simulink model "Coupled3DPathFollowing"  (R2024a)
settings: Solver=ode4  StartTime=0.0  StopTime=inf  FixedStep=0.05  RelTol=1e-3
InitFcn:
  | initModelParam;
  | SetWaypoints;
StopFcn:
  | plotCoupled3DTrack;
values from neighbouring files (symbols this model uses):
  Waypoints = [20 32.5 45 57.5 70 40 63.75 87.5 111.25 135 10 11.25 ... (15 elements, 5x3)]    [Waypoints.mat]
undefined symbols (not defined in the file or in its folder): P0, WPNum
libraries: slpidlib x2, simulink x1, vrlib x1
settings Model: Creator=53549  LastModifiedBy=kedarpandya
settings SolverCC: AlgebraicLoopSolver=TrustRegion
settings DataIOCC: ReturnWorkspaceOutputs=off
settings DebuggingCC: UnconnectedInputMsg=warning  UnconnectedOutputMsg=warning  UnconnectedLineMsg=warning  ArithmeticOperatorsInVariantConditions=warning
settings ModelReferenceCC: EnableRefExpFcnMdlSchedulingChecks=on
settings SFSimCC: SimUseLocalCustomCode=off  CustomCodeUndefinedFunction=UseInterfaceOnly
settings RTWCC: RTWUseLocalCustomCode=off  GPUComputeCapability=3.5  DLArmComputeVersion=19.05
settings CodeAppCC: StateflowObjectComments=on

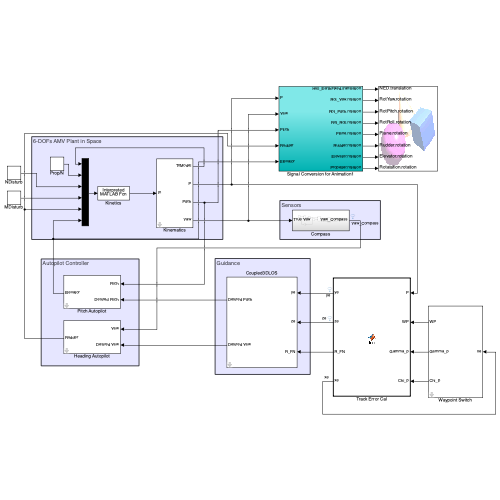
[thumbnail: Simulink's stored preview of the top-level diagram]
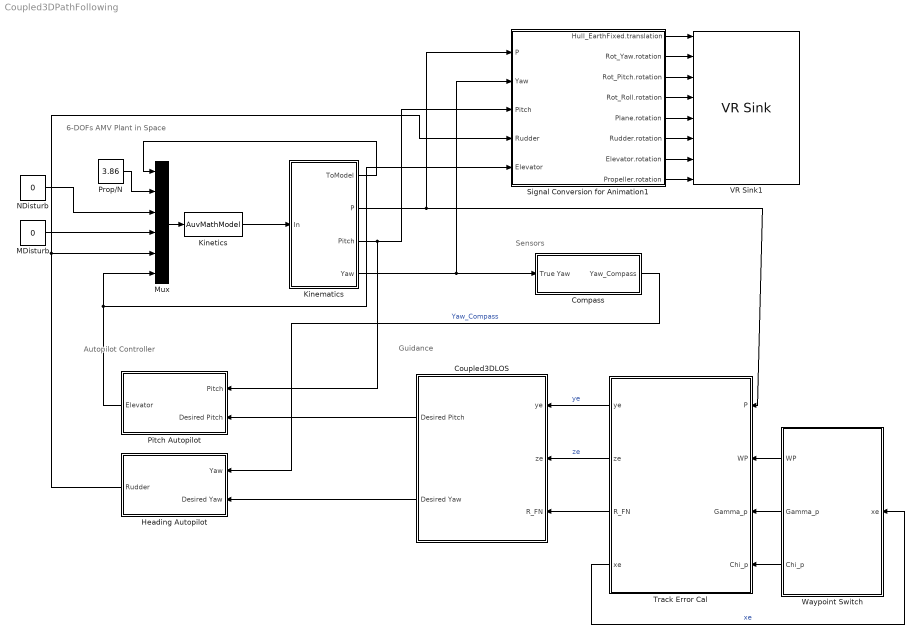
== system Coupled3DPathFollowing ==
  note: Sensors
  note: Guidance
  note: Autopilot Controller
  note: 6-DOFs AMV Plant in Space
  Compass : Subsystem
  Coupled3DLOS : Subsystem  mask{LOSAlg=ALOS, Delta=3, Kapa=0.1, Gamma=0.15}
      mask prompts: LOSAlg "制导算法"; Delta "前视距离"; Kapa "漂角自适应估计增益"; Gamma "攻角自适应估计增益"
      mask TypeOptions LOSAlg: LOS | ALOS
      mask DialogControl DescGroupVar Prompt: 三维视线角制导
      mask DialogControl DescTextVar Prompt: 设置三维视线角制导参数：前视距离，漂角自适应估计增益，漂角自适应估计增益。自适应估计增益设置为0，屏蔽估计补偿；非0，启用估计补偿。
      mask DialogControl Container5 Prompt: 旋转制导算法
      mask DialogControl ParameterGroupVar Prompt: 设置制导参数
  Heading Autopilot : Subsystem  mask{kp=1, ki=0, kd=1.5}
      mask DialogControl DescGroupVar Prompt: Heading Autopilot
      mask DialogControl DescTextVar Prompt: 设置PID增益。
      mask DialogControl ParameterGroupVar Prompt: PID Parameter
  Kinematics : Subsystem  mask{x0=0, y0=0, z0=0.2, pitch0=0, yaw0=68.5, u0=0.6, flowDir=45, flowVel=0.1}
      mask prompts: x0 "Initiral x"; y0 "Initiral y"; z0 "Initiral z"; pitch0 "Initial pitch [Deg]"; yaw0 "Initial yaw [Deg]"; u0 "Initial velocity [m/s]"; flowDir "Flow direction [Deg]"; flowVel "Flow velocity [m/s]"
      mask DialogControl DescGroupVar Prompt: Kinematics
      mask DialogControl DescTextVar Prompt: Set kinematics information: AMV initial state, flow interference, etc
      mask DialogControl ParameterGroupVar Prompt: Initial state
      mask DialogControl Container3 Prompt: Flow
  Kinetics : MATLABFcn  MATLABFcn=AuvMathModel  OutputDimensions=6  OutputSignalType=real
  MDisturb : Constant  Value=0
  Mux : Mux  Inputs=6
  NDisturb : Constant  Value=0
  Pitch Autopilot : Subsystem  mask{kp=2, ki=0.5, kd=1.5}
      mask DialogControl DescGroupVar Prompt: Pitch Autopilot
      mask DialogControl DescTextVar Prompt: 设置PID控制增益。
      mask DialogControl ParameterGroupVar Prompt: PID Parameter
  Prop/N : Constant  Value=3.86
  Signal Conversion for Animation1 : Subsystem
  Track Error Cal : MATLAB Function  TreatAsAtomicUnit=on
  VR Sink1 : vrlib/VR Sink  InstantiateOnLoad=on  SampleTime=0.1  ViewEnable=on  RemoteChange=off  RemoteView=off  FieldsWritten=NED.translation.3.1.1.double#RotYaw.rotation.4.1.1.double#RotPitch.rotation.4.1.1.double#RotRoll.rotation.4.1.1.double#Plane.rotation.4.1.1.double#Rudder.rotation.4.1.1.double#Elevator.rotation.4.1.1.double#Rotatation.rotation.4.1.1.double  WorldFileName=SubMarine.wrl  AutoView=on  VideoDimensions=[]  AllowVariableSize=off  FigureProperties="{'Position', 'Name', 'Viewpoint', 'CameraBound', 'CameraDirection', 'CameraPosition', 'CameraUpVector', 'ZoomFactor', 'Antialiasing', 'Headlight', 'Lighting', 'Sound', 'StatusBar', 'Stereo3D', 'Stereo3DCameraOffset', 'Stereo3DHIT', 'ToolBar', 'Textures', 'Transparency', 'Triad', 'Wireframe', 'NavZones', 'NavMode', 'NavSpeed', 'CaptureFileFormat', 'CaptureFileName', 'Record2DCompressMethod', 'Record2DCompressQuality', 'Record2D', 'Record2DFileName', 'Record2DFPS', 'NavPanel'; [8.6000000000000000e+01   1.0300000000000000e+02   5.7600000000000000e+02   3.5000000000000000e+02], '', 'Stern', 'on', [0.0000000000000000e+00   0.0000000000000000e+00  -1.0000000000000000e+00], [0.0000000000000000e+00   0.0000000000000000e+00   0.0000000000000000e+00], [0.0000000000000000e+00   1.0000000000000000e+00   0.0000000000000000e+00], [1.0000000000000000e+00], 'on', 'on', 'on', 'on', 'on', 'off', [1.0000000149011612e-01], [0.0000000000000000e+00], 'on', 'on', 'on', 'none', 'off', 'off', 'fly', 'normal', 'tif', '%f_anim_%n.tif', 'auto', [7.5000000000000000e+01], 'off', '%f_anim_%n.avi', 'auto', 'halfbar'}"
  Waypoint Switch : Subsystem  mask{WP=Waypoints, WPNum=WPNum}
      mask prompts: WP "航点序列"; WPNum "航点个数"
      mask DialogControl DescGroupVar Prompt: 航点设置
      mask DialogControl DescTextVar Prompt: 设置航点序列和个数
  wires:
  Kinetics/1 -> Kinematics/1(In)
  Mux/1 -> Kinetics/1
  Kinematics/4(Yaw) -> Signal Conversion for Animation1/2(Yaw), Compass/1(True Yaw)
  Kinematics/1(ToModel) -> Mux/1
  Prop/N/1 -> Mux/2
  NDisturb/1 -> Mux/3
  Track Error Cal/4(xe) -> Waypoint Switch/1(xe)  "xe"
  Waypoint Switch/2(Gamma_p) -> Track Error Cal/3(Gamma_p)
  MDisturb/1 -> Mux/4
  Kinematics/2(P) -> Signal Conversion for Animation1/1(P), Track Error Cal/1(P)
  Kinematics/3(Pitch) -> Signal Conversion for Animation1/3(Pitch), Pitch Autopilot/1(Pitch)
  Waypoint Switch/3(Chi_p) -> Track Error Cal/4(Chi_p)
  Waypoint Switch/1(WP) -> Track Error Cal/2(WP)
  Track Error Cal/1(ye) -> Coupled3DLOS/1(ye)  "ye"
  Track Error Cal/2(ze) -> Coupled3DLOS/2(ze)  "ze"
  Track Error Cal/3(R_FN) -> Coupled3DLOS/3(R_FN)
  Coupled3DLOS/1(Desired Pitch) -> Pitch Autopilot/2(Desired Pitch)
  Coupled3DLOS/2(Desired Yaw) -> Heading Autopilot/2(Desired Yaw)
  Compass/1(Yaw_Compass) -> Heading Autopilot/1(Yaw)  "Yaw_Compass"
  Heading Autopilot/1(Rudder) -> Signal Conversion for Animation1/4(Rudder), Mux/5
  Pitch Autopilot/1(Elevator) -> Signal Conversion for Animation1/5(Elevator), Mux/6
  Signal Conversion for Animation1/1(Hull_EarthFixed.translation) -> VR Sink1/1
  Signal Conversion for Animation1/2(Rot_Yaw.rotation) -> VR Sink1/2
  Signal Conversion for Animation1/3(Rot_Pitch.rotation) -> VR Sink1/3
  Signal Conversion for Animation1/4(Rot_Roll.rotation) -> VR Sink1/4
  Signal Conversion for Animation1/5(Plane.rotation) -> VR Sink1/5
  Signal Conversion for Animation1/8(Propeller.rotation) -> VR Sink1/8
  Signal Conversion for Animation1/6(Rudder.rotation) -> VR Sink1/6
  Signal Conversion for Animation1/7(Elevator.rotation) -> VR Sink1/7

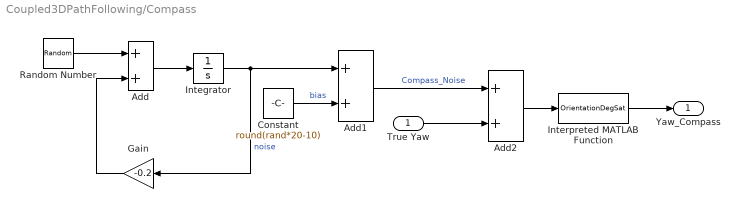
== system Coupled3DPathFollowing/Compass ==
  True Yaw : Inport
  Add : Sum
  Add1 : Sum
  Add2 : Sum
  Constant : Constant  Value=round(rand*20-10)
  Gain : Gain  Gain=-0.2
  Integrator : Integrator
  Interpreted MATLAB Function : MATLABFcn  MATLABFcn=OrientationDegSat
  Random Number : RandomNumber  Variance=0.05  Seed=round(rand*20)  SampleTime=1
  Yaw_Compass : Outport
  wires:
  Constant/1 -> Add1/2  "bias"
  Random Number/1 -> Add/1
  Integrator/1 -> Add1/1, Gain/1  "noise"
  Gain/1 -> Add/2
  Add/1 -> Integrator/1
  Add1/1 -> Add2/1  "Compass_Noise"
  True Yaw/1 -> Add2/2
  Interpreted MATLAB Function/1 -> Yaw_Compass/1
  Add2/1 -> Interpreted MATLAB Function/1

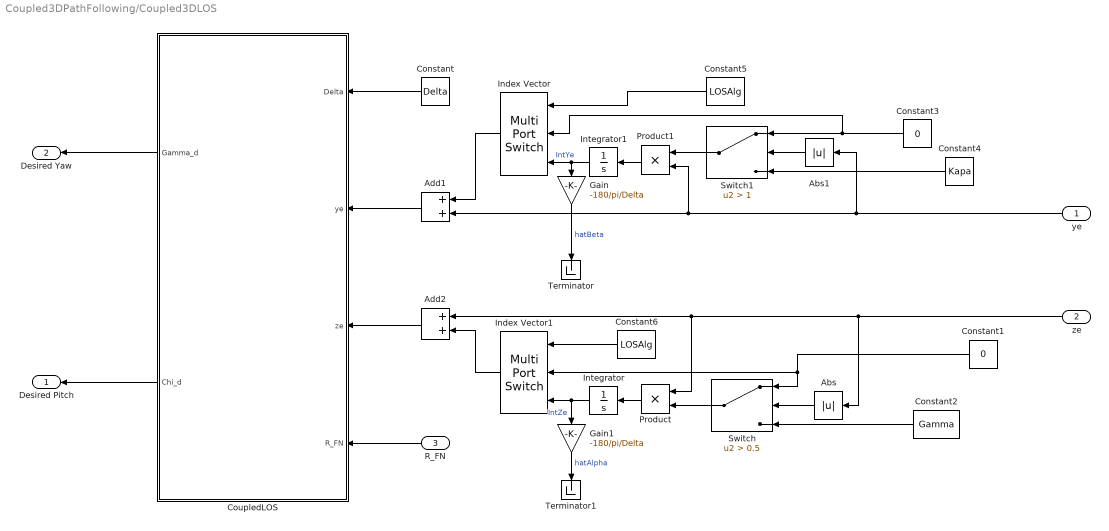
== system Coupled3DPathFollowing/Coupled3DLOS ==
  ye : Inport
  ze : Inport  Port=2
  R_FN : Inport  Port=3
  Abs : Abs  SaturateOnIntegerOverflow=off
  Abs1 : Abs  SaturateOnIntegerOverflow=off
  Add1 : Sum
  Add2 : Sum
  Constant : Constant  Value=Delta
  Constant1 : Constant  Value=0
  Constant2 : Constant  Value=Gamma
  Constant3 : Constant  Value=0
  Constant4 : Constant  Value=Kapa
  Constant5 : Constant  Value=LOSAlg
  Constant6 : Constant  Value=LOSAlg
  CoupledLOS : MATLAB Function  TreatAsAtomicUnit=on
  Gain : Gain  Gain=-180/pi/Delta
  Gain1 : Gain  Gain=-180/pi/Delta
  Index Vector : MultiPortSwitch  Inputs=2  SaturateOnIntegerOverflow=off  InputSameDT=off
  Index Vector1 : MultiPortSwitch  Inputs=2  SaturateOnIntegerOverflow=off  InputSameDT=off
  Integrator : Integrator
  Integrator1 : Integrator
  Product : Product
  Product1 : Product
  Switch : Switch  Criteria=u2 > Threshold  Threshold=0.5  SaturateOnIntegerOverflow=off  InputSameDT=off
  Switch1 : Switch  Criteria=u2 > Threshold  Threshold=1  SaturateOnIntegerOverflow=off  InputSameDT=off
  Terminator : Terminator
  Terminator1 : Terminator
  Desired Pitch : Outport
  Desired Yaw : Outport  Port=2
  wires:
  Abs1/1 -> Switch1/2
  ze/1 -> Abs/1, Add2/1, Product/1
  Constant2/1 -> Switch/3
  Abs/1 -> Switch/2
  Product/1 -> Integrator/1
  Constant4/1 -> Switch1/3
  Constant1/1 -> Index Vector1/2, Switch/1
  ye/1 -> Add1/2, Product1/2, Abs1/1
  Integrator/1 -> Gain1/1, Index Vector1/3  "IntZe"
  Add2/1 -> CoupledLOS/3(ze)
  Product1/1 -> Integrator1/1
  Switch/1 -> Product/2
  Constant/1 -> CoupledLOS/1(Delta)
  CoupledLOS/2(Chi_d) -> Desired Pitch/1
  Switch1/1 -> Product1/1
  Constant3/1 -> Index Vector/2, Switch1/1
  Add1/1 -> CoupledLOS/2(ye)
  CoupledLOS/1(Gamma_d) -> Desired Yaw/1
  Integrator1/1 -> Gain/1, Index Vector/3  "IntYe"
  R_FN/1 -> CoupledLOS/4(R_FN)
  Constant5/1 -> Index Vector/1
  Index Vector/1 -> Add1/1
  Constant6/1 -> Index Vector1/1
  Index Vector1/1 -> Add2/2
  Gain/1 -> Terminator/1  "hatBeta"
  Gain1/1 -> Terminator1/1  "hatAlpha"

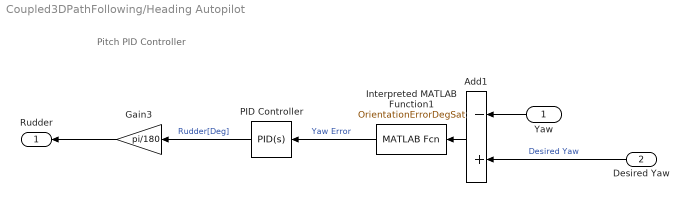
== system Coupled3DPathFollowing/Heading Autopilot ==
  note: Pitch PID Controller
  Yaw : Inport
  Desired Yaw : Inport  Port=2
  Add1 : Sum  Inputs=-+
  Gain3 : Gain  Gain=pi/180
  Interpreted MATLAB Function1 : MATLABFcn  MATLABFcn=OrientationErrorDegSat  OutputDimensions=1
  PID Controller : slpidlib/PID Controller  Controller=PID  Form=Parallel  TimeDomain=Continuous-time  UseExternalTs=off  SampleTime=-1  IntegratorMethod=Forward Euler  FilterMethod=Forward Euler  ControllerParametersSource=internal  P=kp  I=ki  UseKiTs=off  D=kd  UseExternalDerivativeSource=off  N=10  UseFilter=on  TunerSelectOption=Transfer Function Based (PID Tuner App)  InitialConditionSource=internal  InitialConditionForIntegrator=0  InitialConditionForFilter=0  DifferentiatorICPrevScaledInput=0  ExternalReset=none  TrackingMode=off  Kt=1  LimitOutput=on  SatLimitsSource=internal  UpperSaturationLimit=30  LowerSaturationLimit=-30  LinearizeAsGain=on  AntiWindupMode=none  Kb=1  LimitIntegrator=off  UpperIntegratorSaturationLimit=inf  LowerIntegratorSaturationLimit=-inf  POutMin=[]  POutMax=[]  IOutMin=[]  IOutMax=[]  DOutMin=[]  DOutMax=[]  NOutMin=[]  NOutMax=[]  SumOutMin=[]  SumOutMax=[]  SaturationOutMin=[]  SaturationOutMax=[]  PParamMin=[]  PParamMax=[]  IParamMin=[]  IParamMax=[]  DParamMin=[]  DParamMax=[]  NParamMin=[]  NParamMax=[]  KbParamMin=[]  KbParamMax=[]  KtParamMin=[]  KtParamMax=[]  KbOutMin=[]  KbOutMax=[]  KtOutMin=[]  KtOutMax=[]  IntegratorOutMin=[]  IntegratorOutMax=[]  FilterOutMin=[]  FilterOutMax=[]  SumI1OutMin=[]  SumI1OutMax=[]  SumI2OutMin=[]  SumI2OutMax=[]  SumI3OutMin=[]  SumI3OutMax=[]  SumI4OutMin=[]  SumI4OutMax=[]  SumDOutMin=[]  SumDOutMax=[]  DifferentiatorOutMin=[]  DifferentiatorOutMax=[]  FilterDiffOutCoefMin=[]  FilterDiffOutCoefMax=[]  ReciprocalOutMin=[]  ReciprocalOutMax=[]  SumDenOutMin=[]  SumDenOutMax=[]  SumNumOutMin=[]  SumNumOutMax=[]  DivideOutMin=[]  DivideOutMax=[]  UdiffTsProdOutMin=[]  UdiffTsProdOutMax=[]  NTsProdOutMin=[]  NTsProdOutMax=[]  UintegralTsProdOutMin=[]  UintegralTsProdOutMax=[]  UngainTsProdOutMin=[]  UngainTsProdOutMax=[]  ClampingZeroOutDataTypeStr=Inherit: Inherit via back propagation  ClampingZeroOutMin=[]  ClampingZeroOutMax=[]  FilterDenConstantOutDataTypeStr=Inherit: Inherit via back propagation  FilterDenConstantOutMin=[]  FilterDenConstantOutMax=[]  PCopyOutDataTypeStr=Inherit: Inherit via back propagation  PCopyOutMin=[]  PCopyOutMax=[]  NCopyOutDataTypeStr=Inherit: Inherit via back propagation  NCopyOutMin=[]  NCopyOutMax=[]  IntegratorContinuousStateAttributes=''  IntegratorStateMustResolveToSignalObject=off  IntegratorRTWStateStorageClass=Auto  FilterContinuousStateAttributes=''  FilterStateMustResolveToSignalObject=off  FilterRTWStateStorageClass=Auto  ParallelPVariant=InternalParameters  IdealPVariant=Disabled  IVariant=InternalParameters  DVariant=InternalParameters  IntegratorVariant=Continuous  SatVariant=Enabled  AWVariant=Passthrough  PCopyVariant=Disabled  TRVariant=Disabled  FdbkBlocksVariant=Forward  IdealPFdbkVariant=Disabled  SatFdbkVariant=Disabled  DerivativeFilterVariant=ContFilter  NVariant=InternalParameters  NCopyVariant=Disabled  FilterICVariant=InternalICsFilter  IntegratorICVariant=InternalICs  ExternalResetVariant=Disabled  TRSumVariant=Passthrough  SumFdbkVariant=Disabled  SumVariant=Sum_PID  TsampFilterVariant=InternalTs  TsampNgainVariant=Passthrough  TsampIntegralVariant=Disabled_SignalSpec  ExternalSaturationOutDataTypeStr=Inherit: Same as second input  DerivativeSourceVariant=ErrorSignal
  Rudder : Outport
  wires:
  Gain3/1 -> Rudder/1
  Yaw/1 -> Add1/1
  PID Controller/1 -> Gain3/1  "Rudder[Deg]"
  Add1/1 -> Interpreted MATLAB Function1/1
  Desired Yaw/1 -> Add1/2  "Desired Yaw"
  Interpreted MATLAB Function1/1 -> PID Controller/1  "Yaw Error"

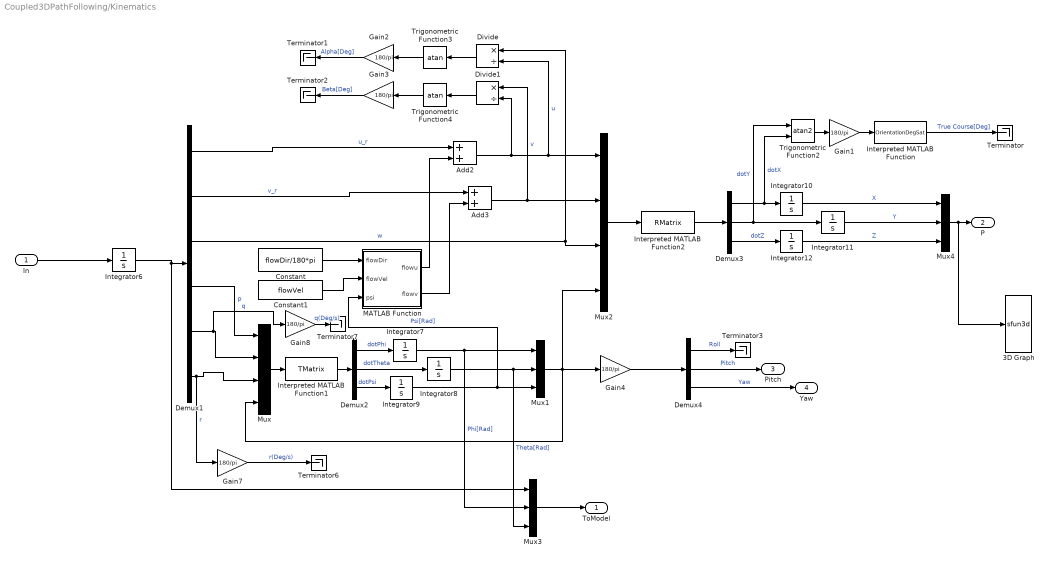
== system Coupled3DPathFollowing/Kinematics ==
  In : Inport
  3D Graph : S-Function  LoadFcn=if exist('sfun3d','file'), sfun3d([],[],[],'LoadBlock'); end  FunctionName=sfun3d  Parameters=ax,T,np,cp,gd,ls,mk,mx,hd,tb  SFunctionDeploymentMode=off  EnableBusSupport=off  mask(3D Graph){np=1, ax=[-100 100 -20 300 -5 20], mx=1e4, T=0.1, cp=[3 2 1], gd=on, hd=off, tb=off, ls=-, mk=none}
      mask prompts: np "Number of moving points (lines)"; ax "Range: [xmin xmax  ymin ymax zmin zmax]"; mx "Max number of points in each line"; T "Sampling Time"; cp "Camera position (use [0 0 1] for 2D XY view)"; gd "Grid (on|off)"; hd "HeadMarkers (on|off)"; tb "Toolbar (on|off)"; ls "LineStyle"; mk "LineMarker"
      mask help:
      | This block plots the position of several points in the XYZ space. The input contains the coordinates of all the points (x1,y1,z1,x2,y2,z2,...).
      | The number of moving points (lines), the XYZ ranges, sampling time, camera position, and grid (among other things) can be set as mask parameters.
      settings: CopyFcn=if exist('sfun3d','file'), sfun3d([],[],[],'CopyBlock'); end  DeleteFcn=if exist('sfun3d','file'), sfun3d([],[],[],'DeleteBlock'); end  NameChangeFcn=if exist('sfun3d','file'), sfun3d([],[],[],'NameChange'); end
      mask Help:
      | This block plots the position of several points in the XYZ space. The input contains the coordinates of all the points (x1,y1,z1,x2,y2,z2,...).
      | The number of moving points (lines), the XYZ ranges, sampling time, camera position, and grid (among other things) can be set as mask parameters.
      mask TypeOptions ls: - | -- | : | -. | none
      mask TypeOptions mk: none | . | + | o | * | x | square | diamond | v | ^ | > | < | pentagram | hexagram
      mask Display: plot([.05 .95 .95 .05 .05],[.45 .45 .95 .95 .45], 0.5+cos(0:0.1:2*pi)*0.3,0.7+sin(0:0.1:2*pi)*0.2)
  Add2 : Sum
  Add3 : Sum
  Constant : Constant  Value=flowDir/180*pi
  Constant1 : Constant  Value=flowVel
  Demux1 : Demux  Outputs=6
  Demux2 : Demux  Outputs=3
  Demux3 : Demux  Outputs=3
  Demux4 : Demux  Outputs=3
  Divide : Product  Inputs=*/
  Divide1 : Product  Inputs=*/
  Gain{1..4,7..8} (6 alike) : Gain  Gain=180/pi
  Integrator10 : Integrator  InitialCondition=x0
  Integrator11 : Integrator  InitialCondition=y0
  Integrator12 : Integrator  InitialCondition=z0
  Integrator6 : Integrator  InitialCondition=[u0; 0; 0; 0; 0; 0]
  Integrator7 : Integrator
  Integrator8 : Integrator  InitialCondition=pitch0/180*pi
  Integrator9 : Integrator  InitialCondition=yaw0*pi/180  WrapState=on  WrappedStateUpperValue=6.2832  WrappedStateLowerValue=0
  Interpreted MATLAB Function : MATLABFcn  MATLABFcn=OrientationDegSat
  Interpreted MATLAB Function1 : MATLABFcn  MATLABFcn=TMatrix  OutputDimensions=3
  Interpreted MATLAB Function2 : MATLABFcn  MATLABFcn=RMatrix  OutputDimensions=3
  MATLAB Function : MATLAB Function  TreatAsAtomicUnit=on
  Mux : Mux
  Mux1 : Mux  Inputs=3
  Mux2 : Mux
  Mux3 : Mux  Inputs=3
  Mux4 : Mux  Inputs=3
  Terminator{,1..3,6..7} (6 alike) : Terminator
  Trigonometric Function2 : Trigonometry  Operator=atan2
  Trigonometric Function3 : Trigonometry  Operator=atan
  Trigonometric Function4 : Trigonometry  Operator=atan
  ToModel : Outport
  P : Outport  Port=2
  Pitch : Outport  Port=3
  Yaw : Outport  Port=4
  wires:
  Constant/1 -> MATLAB Function/1(flowDir)
  Constant1/1 -> MATLAB Function/2(flowVel)
  Integrator6/1 -> Mux3/1, Demux1/1
  Demux1/4 -> Mux/1  "p"
  Demux1/5 -> Gain8/1, Mux/2  "q"
  Demux1/6 -> Gain7/1, Mux/3  "r"
  Mux/1 -> Interpreted MATLAB Function1/1
  Interpreted MATLAB Function1/1 -> Demux2/1
  Demux2/1 -> Integrator7/1  "dotPhi"
  Demux2/2 -> Integrator8/1  "dotTheta"
  Demux2/3 -> Integrator9/1  "dotPsi"
  Integrator9/1 -> MATLAB Function/3(psi), Mux1/3  "Psi[Rad]"
  Integrator7/1 -> Mux1/1, Mux3/2  "Phi[Rad]"
  Integrator8/1 -> Mux3/3, Mux1/2  "Theta[Rad]"
  Mux1/1 -> Gain4/1, Mux/4, Mux2/4
  Demux1/1 -> Add2/1  "u_r"
  Demux1/2 -> Add3/1  "v_r"
  Demux1/3 -> Mux2/3, Divide/1  "w"
  Mux2/1 -> Interpreted MATLAB Function2/1
  Interpreted MATLAB Function2/1 -> Demux3/1
  Demux3/1 -> Trigonometric Function2/2, Integrator10/1  "dotX"
  Demux3/2 -> Trigonometric Function2/1, Integrator11/1  "dotY"
  Demux3/3 -> Integrator12/1  "dotZ"
  Integrator10/1 -> Mux4/1  "X"
  Integrator11/1 -> Mux4/2  "Y"
  Integrator12/1 -> Mux4/3  "Z"
  Gain2/1 -> Terminator1/1  "Alpha[Deg]"
  Trigonometric Function3/1 -> Gain2/1
  Divide/1 -> Trigonometric Function3/1
  Divide1/1 -> Trigonometric Function4/1
  Trigonometric Function4/1 -> Gain3/1
  Gain3/1 -> Terminator2/1  "Beta[Deg]"
  Gain1/1 -> Interpreted MATLAB Function/1
  Interpreted MATLAB Function/1 -> Terminator/1  "True Course[Deg]"
  Trigonometric Function2/1 -> Gain1/1
  Add2/1 -> Divide1/2, Divide/2, Mux2/1  "u"
  Add3/1 -> Mux2/2, Divide1/1  "v"
  MATLAB Function/1(flowu) -> Add2/2
  MATLAB Function/2(flowv) -> Add3/2
  Gain4/1 -> Demux4/1
  Demux4/1 -> Terminator3/1  "Roll"
  Demux4/2 -> Pitch/1  "Pitch"
  Demux4/3 -> Yaw/1  "Yaw"
  Mux3/1 -> ToModel/1
  Mux4/1 -> 3D Graph/1, P/1
  In/1 -> Integrator6/1
  Gain7/1 -> Terminator6/1  "r(Deg/s)"
  Gain8/1 -> Terminator7/1  "q(Deg/s)"

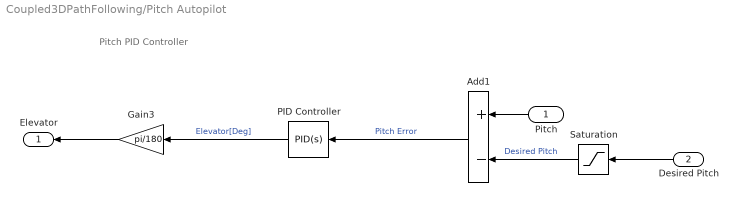
== system Coupled3DPathFollowing/Pitch Autopilot ==
  note: Pitch PID Controller
  Pitch : Inport
  Desired Pitch : Inport  Port=2
  Add1 : Sum  Inputs=+-
  Gain3 : Gain  Gain=pi/180
  PID Controller : slpidlib/PID Controller  Controller=PID  Form=Parallel  TimeDomain=Continuous-time  UseExternalTs=off  SampleTime=-1  IntegratorMethod=Forward Euler  FilterMethod=Forward Euler  ControllerParametersSource=internal  P=kp  I=ki  UseKiTs=off  D=kd  UseExternalDerivativeSource=off  N=10  UseFilter=on  TunerSelectOption=Transfer Function Based (PID Tuner App)  InitialConditionSource=internal  InitialConditionForIntegrator=0  InitialConditionForFilter=0  DifferentiatorICPrevScaledInput=0  ExternalReset=none  TrackingMode=off  Kt=1  LimitOutput=on  SatLimitsSource=internal  UpperSaturationLimit=30  LowerSaturationLimit=-30  LinearizeAsGain=on  AntiWindupMode=none  Kb=1  LimitIntegrator=off  UpperIntegratorSaturationLimit=inf  LowerIntegratorSaturationLimit=-inf  POutMin=[]  POutMax=[]  IOutMin=[]  IOutMax=[]  DOutMin=[]  DOutMax=[]  NOutMin=[]  NOutMax=[]  SumOutMin=[]  SumOutMax=[]  SaturationOutMin=[]  SaturationOutMax=[]  PParamMin=[]  PParamMax=[]  IParamMin=[]  IParamMax=[]  DParamMin=[]  DParamMax=[]  NParamMin=[]  NParamMax=[]  KbParamMin=[]  KbParamMax=[]  KtParamMin=[]  KtParamMax=[]  KbOutMin=[]  KbOutMax=[]  KtOutMin=[]  KtOutMax=[]  IntegratorOutMin=[]  IntegratorOutMax=[]  FilterOutMin=[]  FilterOutMax=[]  SumI1OutMin=[]  SumI1OutMax=[]  SumI2OutMin=[]  SumI2OutMax=[]  SumI3OutMin=[]  SumI3OutMax=[]  SumI4OutMin=[]  SumI4OutMax=[]  SumDOutMin=[]  SumDOutMax=[]  DifferentiatorOutMin=[]  DifferentiatorOutMax=[]  FilterDiffOutCoefMin=[]  FilterDiffOutCoefMax=[]  ReciprocalOutMin=[]  ReciprocalOutMax=[]  SumDenOutMin=[]  SumDenOutMax=[]  SumNumOutMin=[]  SumNumOutMax=[]  DivideOutMin=[]  DivideOutMax=[]  UdiffTsProdOutMin=[]  UdiffTsProdOutMax=[]  NTsProdOutMin=[]  NTsProdOutMax=[]  UintegralTsProdOutMin=[]  UintegralTsProdOutMax=[]  UngainTsProdOutMin=[]  UngainTsProdOutMax=[]  ClampingZeroOutDataTypeStr=Inherit: Inherit via back propagation  ClampingZeroOutMin=[]  ClampingZeroOutMax=[]  FilterDenConstantOutDataTypeStr=Inherit: Inherit via back propagation  FilterDenConstantOutMin=[]  FilterDenConstantOutMax=[]  PCopyOutDataTypeStr=Inherit: Inherit via back propagation  PCopyOutMin=[]  PCopyOutMax=[]  NCopyOutDataTypeStr=Inherit: Inherit via back propagation  NCopyOutMin=[]  NCopyOutMax=[]  IntegratorContinuousStateAttributes=''  IntegratorStateMustResolveToSignalObject=off  IntegratorRTWStateStorageClass=Auto  FilterContinuousStateAttributes=''  FilterStateMustResolveToSignalObject=off  FilterRTWStateStorageClass=Auto  ParallelPVariant=InternalParameters  IdealPVariant=Disabled  IVariant=InternalParameters  DVariant=InternalParameters  IntegratorVariant=Continuous  SatVariant=Enabled  AWVariant=Passthrough  PCopyVariant=Disabled  TRVariant=Disabled  FdbkBlocksVariant=Forward  IdealPFdbkVariant=Disabled  SatFdbkVariant=Disabled  DerivativeFilterVariant=ContFilter  NVariant=InternalParameters  NCopyVariant=Disabled  FilterICVariant=InternalICsFilter  IntegratorICVariant=InternalICs  ExternalResetVariant=Disabled  TRSumVariant=Passthrough  SumFdbkVariant=Disabled  SumVariant=Sum_PID  TsampFilterVariant=InternalTs  TsampNgainVariant=Passthrough  TsampIntegralVariant=Disabled_SignalSpec  ExternalSaturationOutDataTypeStr=Inherit: Same as second input  DerivativeSourceVariant=ErrorSignal
  Saturation : Saturate  UpperLimit=25  LowerLimit=-25
  Elevator : Outport
  wires:
  Add1/1 -> PID Controller/1  "Pitch Error"
  Desired Pitch/1 -> Saturation/1
  PID Controller/1 -> Gain3/1  "Elevator[Deg]"
  Pitch/1 -> Add1/1
  Gain3/1 -> Elevator/1
  Saturation/1 -> Add1/2  "Desired Pitch"

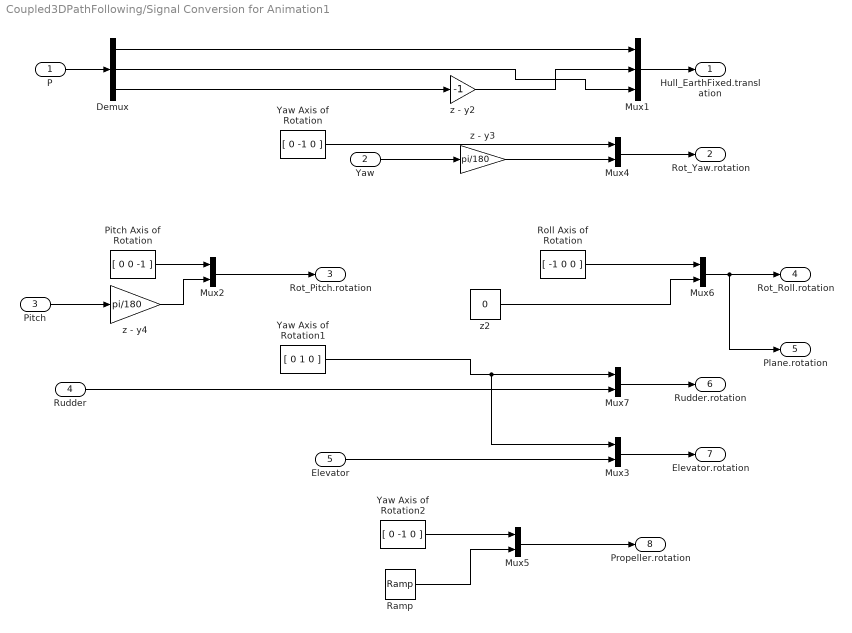
== system Coupled3DPathFollowing/Signal Conversion for Animation1 ==
  P : Inport
  Yaw : Inport  Port=2
  Pitch : Inport  Port=3
  Rudder : Inport  Port=4
  Elevator : Inport  Port=5
  Demux : Demux  Outputs=3
  Mux1 : Mux  Inputs=3
  Mux{2..7} (6 alike) : Mux  Inputs=2
  Pitch Axis of Rotation : Constant  Value=[ 0 0 -1 ]
  Ramp : simulink/Sources/Ramp  slope=2  start=0  InitialOutput=0
  Roll Axis of Rotation : Constant  Value=[ -1 0 0 ]
  Yaw Axis of Rotation : Constant  Value=[ 0 -1 0 ]
  Yaw Axis of Rotation1 : Constant  Value=[ 0 1 0 ]
  Yaw Axis of Rotation2 : Constant  Value=[ 0 -1 0 ]
  z - y2 : Gain  Gain=-1
  z - y3 : Gain  Gain=pi/180
  z - y4 : Gain  Gain=pi/180
  z2 : Constant  Value=0
  Hull_EarthFixed.translation : Outport
  Rot_Yaw.rotation : Outport  Port=2
  Rot_Pitch.rotation : Outport  Port=3
  Rot_Roll.rotation : Outport  Port=4
  Plane.rotation : Outport  Port=5
  Rudder.rotation : Outport  Port=6
  Elevator.rotation : Outport  Port=7
  Propeller.rotation : Outport  Port=8
  wires:
  Roll Axis of Rotation/1 -> Mux6/1
  z2/1 -> Mux6/2
  Demux/3 -> z - y2/1
  z - y2/1 -> Mux1/2
  Demux/2 -> Mux1/3
  Yaw Axis of Rotation/1 -> Mux4/1
  Mux1/1 -> Hull_EarthFixed.translation/1
  P/1 -> Demux/1
  Rudder/1 -> Mux7/2
  Mux7/1 -> Rudder.rotation/1
  Mux4/1 -> Rot_Yaw.rotation/1
  Mux6/1 -> Plane.rotation/1, Rot_Roll.rotation/1
  Yaw/1 -> z - y3/1
  Pitch Axis of Rotation/1 -> Mux2/1
  Mux2/1 -> Rot_Pitch.rotation/1
  z - y4/1 -> Mux2/2
  Pitch/1 -> z - y4/1
  Demux/1 -> Mux1/1
  z - y3/1 -> Mux4/2
  Yaw Axis of Rotation1/1 -> Mux3/1, Mux7/1
  Mux3/1 -> Elevator.rotation/1
  Elevator/1 -> Mux3/2
  Yaw Axis of Rotation2/1 -> Mux5/1
  Mux5/1 -> Propeller.rotation/1
  Ramp/1 -> Mux5/2

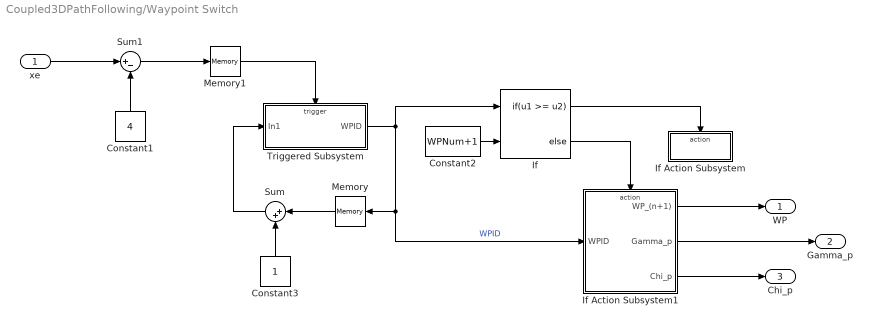
== system Coupled3DPathFollowing/Waypoint Switch ==
  xe : Inport
  Constant1 : Constant  Value=4
  Constant2 : Constant  Value=WPNum+1
  Constant3 : Constant
  If : If  NumInputs=2  IfExpression=u1 >= u2
  If Action Subsystem : Subsystem  TreatAsAtomicUnit=on
  If Action Subsystem1 : Subsystem  TreatAsAtomicUnit=on
  Memory : Memory  InitialCondition=1  InheritSampleTime=on
  Memory1 : Memory  InitialCondition=5  InheritSampleTime=on
  Sum : Sum  Inputs=|++
  Sum1 : Sum  Inputs=|+-
  Triggered Subsystem : Subsystem  TreatAsAtomicUnit=on
  WP : Outport
  Gamma_p : Outport  Port=2
  Chi_p : Outport  Port=3
  wires:
  Constant2/1 -> If/2
  If Action Subsystem1/2(Gamma_p) -> Gamma_p/1
  Sum1/1 -> Memory1/1
  Memory/1 -> Sum/1
  If/2 -> If Action Subsystem1/Action
  xe/1 -> Sum1/1
  Sum/1 -> Triggered Subsystem/1(In1)
  Constant3/1 -> Sum/2
  If Action Subsystem1/1(WP_(n+1)) -> WP/1
  Triggered Subsystem/1(WPID) -> If/1, If Action Subsystem1/1(WPID), Memory/1  "WPID"
  Constant1/1 -> Sum1/2
  If/1 -> If Action Subsystem/Action
  Memory1/1 -> Triggered Subsystem/Trigger
  If Action Subsystem1/3(Chi_p) -> Chi_p/1

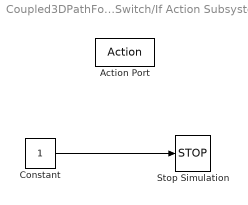
== system Coupled3DPathFollowing/Waypoint Switch/If Action Subsystem ==
  Action Port : ActionPort  ActionPortLabel=if(u1 >= u2)
  Constant : Constant
  Stop Simulation : Stop
  wires:
  Constant/1 -> Stop Simulation/1

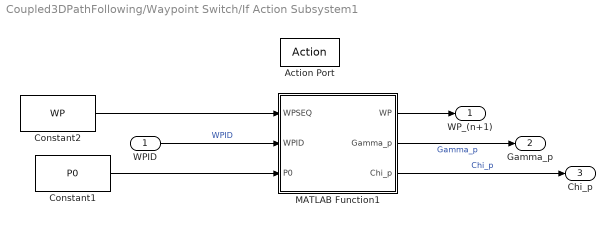
== system Coupled3DPathFollowing/Waypoint Switch/If Action Subsystem1 ==
  WPID : Inport
  Action Port : ActionPort  ActionPortLabel=else
  Constant1 : Constant  Value=P0
  Constant2 : Constant  Value=WP
  MATLAB Function1 : MATLAB Function  TreatAsAtomicUnit=on
  WP_(n+1) : Outport
  Gamma_p : Outport  Port=2
  Chi_p : Outport  Port=3
  wires:
  MATLAB Function1/2(Gamma_p) -> Gamma_p/1  "Gamma_p"
  MATLAB Function1/1(WP) -> WP_(n+1)/1
  Constant2/1 -> MATLAB Function1/1(WPSEQ)
  WPID/1 -> MATLAB Function1/2(WPID)  "WPID"
  MATLAB Function1/3(Chi_p) -> Chi_p/1  "Chi_p"
  Constant1/1 -> MATLAB Function1/3(P0)

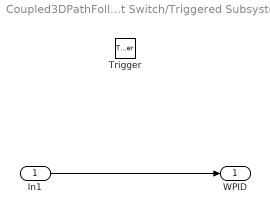
== system Coupled3DPathFollowing/Waypoint Switch/Triggered Subsystem ==
  In1 : Inport
  Trigger : TriggerPort  TriggerType=falling  VariantControl=Variant
  WPID : Outport  InitialOutput=1
  wires:
  In1/1 -> WPID/1

== matlab function Coupled3DPathFollowing/Waypoint Switch/If Action Subsystem1/MATLAB Function1 ==
  data: WP output; WPSEQ input; WPID input; Gamma_p output; Chi_p output; P0 input
function [WP,Gamma_p,Chi_p] = fcn(WPSEQ,WPID,P0)
WP = WPSEQ(WPID,:)';

if WPID == 1
    dx = WPSEQ(1,1)-P0(1);dy = WPSEQ(1,2)-P0(2);dz = WPSEQ(1,3)-P0(3);
else
    dp = WPSEQ(WPID,:)-WPSEQ(WPID-1,:);
    dx = dp(1);dy = dp(2);dz = dp(3);
end

Gamma_p = atan2(dy,dx);
Chi_p = -atan(dz/sqrt(dx*dx+dy*dy));

if Gamma_p<0
    Gamma_p = Gamma_p + 2*pi;
end

== matlab function Coupled3DPathFollowing/Track Error Cal ==
  data: ye output; ze output; P input; WP input; Gamma_p input; Chi_p input; R_FN output; xe output
function [ye,ze,R_FN,xe] = fcn(P,WP,Gamma_p,Chi_p)
sg = sin(Gamma_p);cg = cos(Gamma_p);
sc = sin(Chi_p);cc = cos(Chi_p);
R_FN = [cg*cc -sg cg*sc; sg*cc cg sg*sc; -sc 0 cc];
R_NF = R_FN';
E_F = R_NF*(WP-P);

xe = E_F(1);
ye = E_F(2);
ze = E_F(3);
end

== matlab function Coupled3DPathFollowing/Kinematics/MATLAB Function ==
  data: flowDir input; flowu output; flowVel input; psi input; flowv output
function [flowu,flowv] = fcn(flowDir,flowVel,psi)
dAngle = flowDir - psi;
if dAngle > 2*pi
    dAngle = dAngle-2*pi;
elseif dAngle<0
    dAngle = dAngle+2*pi;
end
flowu = flowVel*cos(dAngle);
flowv = flowVel*sin(dAngle);

== matlab function Coupled3DPathFollowing/Coupled3DLOS/CoupledLOS ==
  data: Gamma_d output; Chi_d output; Delta input; ye input; ze input; R_FN input
function [Gamma_d,Chi_d] = fcn(Delta,ye,ze,R_FN)

LOS_F = [Delta;ye;ze];
LOS_N = R_FN*LOS_F;
Gamma_d = atan2(LOS_N(2),LOS_N(1));
%Gamma_d = atan2(LOS_N(2),sign(LOS_N(1))*sqrt(LOS_N(1)*LOS_N(1)+LOS_N(3)*LOS_N(3)));
if Gamma_d<0
    Gamma_d = Gamma_d+2*pi;
end
Gamma_d = Gamma_d*180/pi;
Chi_d = -atan(LOS_N(3)/sqrt(LOS_N(1)^2+LOS_N(2)^2))*180/pi;
%Chi_d = -atan(LOS_N(3)/abs(LOS_N(1)))*180/pi;
end
